simulink model "Harness_computeBaseFourierSubset"  (R2017b)
settings: Solver=FixedStepDiscrete  StartTime=0.0  StopTime=simulationTime/3  RelTol=1e-3
InitFcn:
  | referenceVector = getBaseFourierSubset(nRecurrences, nFilters);
undefined symbols (not defined in the file): nFilters, oversamplingFactor, sizeRAMs
settings Model: Creator=pnowodzi  LastModifiedBy=pnowodzi
settings DataIOCC: ExternalInput=tb_computeBaseFourierSubset.getElement('phaseIncrement'),tb_computeBaseFourierSubset.getElement('startAnalysis'),tb_computeBaseFourierSubset.getElement('syncRecurrence'),tb_computeBaseFourierSubset.getElement('nRecurrences')  LimitDataPoints=on  LoadExternalInput=on  SaveTime=off
settings OptimizationCC: BlockReduction=off  ConditionallyExecuteInputs=off  DefaultParameterBehavior=Inlined  LifeSpan=inf
settings DebuggingCC: AlgebraicLoopMsg=error  SingleTaskRateTransMsg=error  AllowSymbolicDim=off  StrictBusMsg=ErrorOnBusTreatedAsVector  SFUnexpectedBacktrackingDiag=warning  SFNoUnconditionalDefaultTransitionDiag=warning  SFExecutionAtInitializationDiag=none
settings HardwareCC: ProdBitPerPointer=32  ProdBitPerSizeT=32  ProdBitPerPtrDiffT=32  ProdLargestAtomicFloat=None  ProdIntDivRoundTo=Undefined  ProdEndianess=Unspecified  ProdWordSize=32  ProdHWDeviceType=ASIC/FPGA->ASIC/FPGA  ProdEqTarget=off
settings CodeAppCC: StateflowObjectComments=on
settings GRTTargetCC: TargetLangStandard=C89/C90 (ANSI)  GeneratePreprocessorConditionals=Disable all
settings ConfigComp: CovScope=ReferencedModels  CovMetricSettings=dw  CovHtmlReporting=on  CovSaveCumulativeToWorkspaceVar=on  CovSaveSingleToWorkspaceVar=on  CovExternalEMLEnable=off  CovSFcnEnable=off

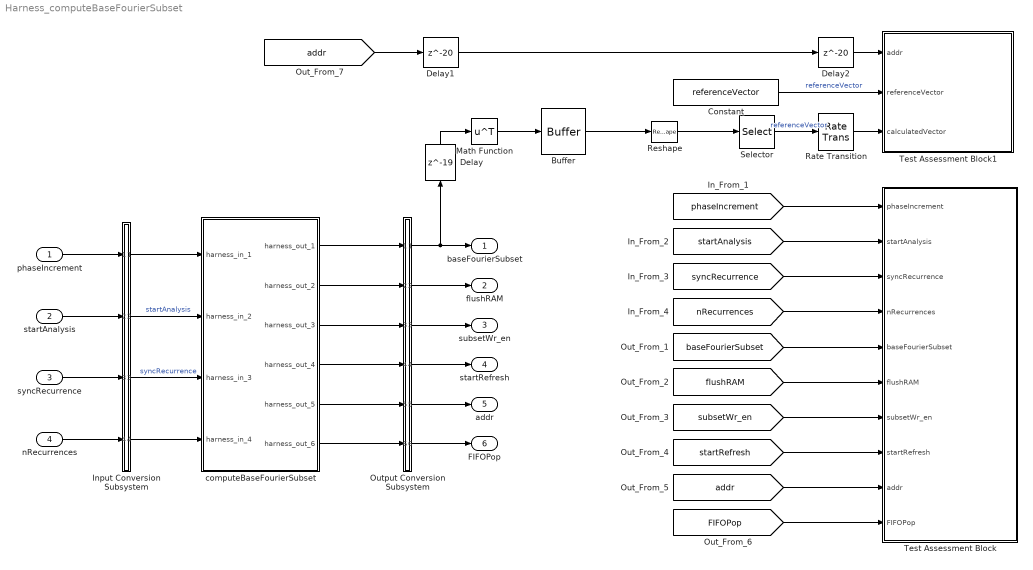
== system Harness_computeBaseFourierSubset ==
  phaseIncrement : Inport  OutDataTypeStr=fixdt('ufix16_En20')  PortDimensions=[1]  SampleTime=4e-09  Interpolate=off
  startAnalysis : Inport  Port=2  OutDataTypeStr=boolean  PortDimensions=[1]  SampleTime=4e-09
  syncRecurrence : Inport  Port=3  OutDataTypeStr=boolean  PortDimensions=[1]  SampleTime=4e-09
  nRecurrences : Inport  Port=4  OutDataTypeStr=fixdt('ufix10')  PortDimensions=[1]  SampleTime=4e-09  Interpolate=off
  Buffer : Buffer  N=oversamplingFactor  OutputFrames=off
  Constant : Constant  Value=referenceVector  SampleTime=-1
  Delay : Delay  DelayLength=19
  Delay1 : Delay  DelayLength=20
  Delay2 : Delay  DelayLength=20
  Input Conversion Subsystem : Subsystem  Tag=__SLT_ICS__  Description=|
      | Signal spec.
      | and routing
      settings: AttributesFormatString=%<Description>
  Math Function : Math  Operator=transpose  SaturateOnIntegerOverflow=on
  Output Conversion Subsystem : Subsystem  Tag=__SLT_OCS__  Description=|
      | Signal spec.
      | and routing
      settings: AttributesFormatString=%<Description>
  Rate Transition : RateTransition
  Reshape : Reshape
  Selector : Selector  InputPortWidth=ceil(nFilters/2/oversamplingFactor)*oversamplingFactor  IndexOptions=Index vector (dialog)  Indices=(1:floor((nFilters-1)/2 + 1))  OutputSizes=1
  Test Assessment Block : Test Sequence  Tag=__SLT_ASMT__  TreatAsAtomicUnit=on
  Test Assessment Block1 : Test Sequence  Tag=__SLT_ASMT__  TreatAsAtomicUnit=on
  computeBaseFourierSubset : Subsystem  Tag=__SL_testing_harness_stub_
  baseFourierSubset : Outport  OutDataTypeStr=single  PortDimensions=[6, 1]
      settings: SignalType=complex
  flushRAM : Outport  Port=2  OutDataTypeStr=boolean  PortDimensions=[1]
  subsetWr_en : Outport  Port=3  OutDataTypeStr=boolean  PortDimensions=[1]
  startRefresh : Outport  Port=4  OutDataTypeStr=boolean  PortDimensions=[1]
  addr : Outport  Port=5  OutDataTypeStr=uint8  PortDimensions=[1]
  FIFOPop : Outport  Port=6  OutDataTypeStr=boolean  PortDimensions=[1]
  wires:
  [phaseIncrement] -> Test Assessment Block/1(phaseIncrement)
  [startAnalysis] -> Test Assessment Block/2(startAnalysis)
  [syncRecurrence] -> Test Assessment Block/3(syncRecurrence)
  [nRecurrences] -> Test Assessment Block/4(nRecurrences)
  [baseFourierSubset] -> Test Assessment Block/5(baseFourierSubset)
  [flushRAM] -> Test Assessment Block/6(flushRAM)
  [subsetWr_en] -> Test Assessment Block/7(subsetWr_en)
  [startRefresh] -> Test Assessment Block/8(startRefresh)
  [addr] -> Test Assessment Block/9(addr)
  [FIFOPop] -> Test Assessment Block/10(FIFOPop)
  phaseIncrement/1 -> Input Conversion Subsystem/1(Inport_1)
  startAnalysis/1 -> Input Conversion Subsystem/2(Inport_2)
  syncRecurrence/1 -> Input Conversion Subsystem/3(Inport_3)
  Output Conversion Subsystem/1(Outport_1) -> Delay/1, baseFourierSubset/1
  Output Conversion Subsystem/2(Outport_2) -> flushRAM/1
  Output Conversion Subsystem/3(Outport_3) -> subsetWr_en/1
  Output Conversion Subsystem/4(Outport_4) -> startRefresh/1
  Output Conversion Subsystem/5(Outport_5) -> addr/1
  Output Conversion Subsystem/6(Outport_6) -> FIFOPop/1
  Input Conversion Subsystem/1(Outport_1) -> computeBaseFourierSubset/1(harness_in_1)
  Input Conversion Subsystem/2(Outport_2) -> computeBaseFourierSubset/2(harness_in_2)  "startAnalysis"
  Input Conversion Subsystem/3(Outport_3) -> computeBaseFourierSubset/3(harness_in_3)  "syncRecurrence"
  Input Conversion Subsystem/4(Outport_4) -> computeBaseFourierSubset/4(harness_in_4)
  computeBaseFourierSubset/1(harness_out_1) -> Output Conversion Subsystem/1(Inport_1)
  computeBaseFourierSubset/2(harness_out_2) -> Output Conversion Subsystem/2(Inport_2)
  computeBaseFourierSubset/3(harness_out_3) -> Output Conversion Subsystem/3(Inport_3)
  computeBaseFourierSubset/4(harness_out_4) -> Output Conversion Subsystem/4(Inport_4)
  computeBaseFourierSubset/6(harness_out_6) -> Output Conversion Subsystem/6(Inport_6)
  Reshape/1 -> Selector/1
  nRecurrences/1 -> Input Conversion Subsystem/4(Inport_4)
  Constant/1 -> Test Assessment Block1/2(referenceVector)  "referenceVector"
  Math Function/1 -> Buffer/1
  Delay/1 -> Math Function/1
  Buffer/1 -> Reshape/1
  Selector/1 -> Rate Transition/1  "referenceVector"
  [addr] -> Delay1/1
  computeBaseFourierSubset/5(harness_out_5) -> Output Conversion Subsystem/5(Inport_5)
  Delay1/1 -> Delay2/1
  Rate Transition/1 -> Test Assessment Block1/3(calculatedVector)
  Delay2/1 -> Test Assessment Block1/1(addr)

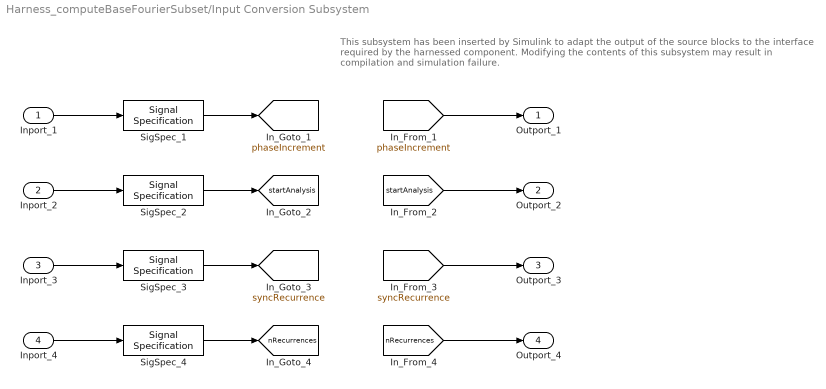
== system Harness_computeBaseFourierSubset/Input Conversion Subsystem ==
  note: This subsystem has been inserted by Simulink to adapt the output of the source blocks to the interface required by the harnessed component.
      |  Modifying the contents of this subsystem may result in compilation and simulation failure.
  Inport_1 : Inport
  Inport_2 : Inport  Port=2
  Inport_3 : Inport  Port=3
  Inport_4 : Inport  Port=4
  SigSpec_1 : SignalSpecification  OutDataTypeStr=fixdt('ufix16_En20')  Dimensions=[1]  SampleTime=4e-09
  SigSpec_2 : SignalSpecification  OutDataTypeStr=boolean  Dimensions=[1]  SampleTime=4e-09
  SigSpec_3 : SignalSpecification  OutDataTypeStr=boolean  Dimensions=[1]  SampleTime=4e-09
  SigSpec_4 : SignalSpecification  OutDataTypeStr=fixdt('ufix10')  Dimensions=[1]  SampleTime=4e-09
  Outport_1 : Outport
  Outport_2 : Outport  Port=2
  Outport_3 : Outport  Port=3
  Outport_4 : Outport  Port=4
  tag scope: nRecurrences=global, phaseIncrement=global, startAnalysis=global, syncRecurrence=global
  wires:
  [phaseIncrement] -> Outport_1/1
  SigSpec_1/1 -> [phaseIncrement]
  Inport_1/1 -> SigSpec_1/1
  [startAnalysis] -> Outport_2/1
  SigSpec_2/1 -> [startAnalysis]
  Inport_2/1 -> SigSpec_2/1
  [syncRecurrence] -> Outport_3/1
  SigSpec_3/1 -> [syncRecurrence]
  Inport_3/1 -> SigSpec_3/1
  [nRecurrences] -> Outport_4/1
  SigSpec_4/1 -> [nRecurrences]
  Inport_4/1 -> SigSpec_4/1

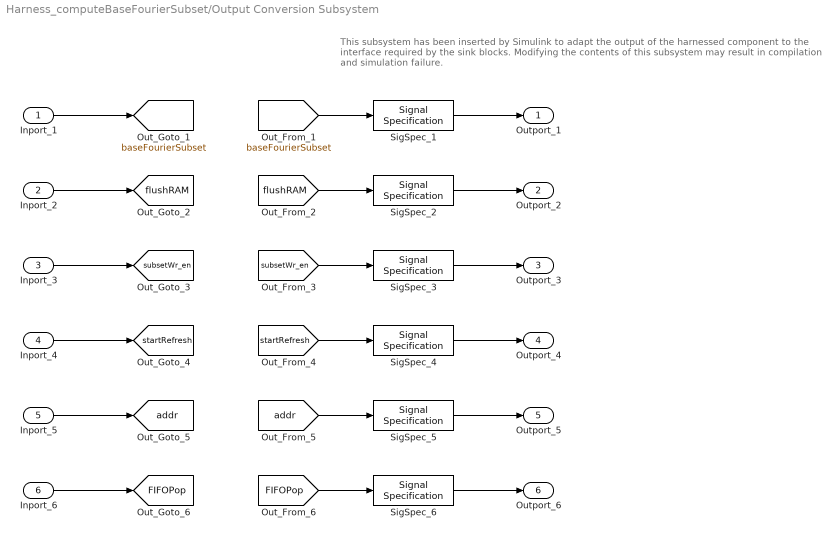
== system Harness_computeBaseFourierSubset/Output Conversion Subsystem ==
  note: This subsystem has been inserted by Simulink to adapt the output of the harnessed component to the interface required by the sink blocks.
      |  Modifying the contents of this subsystem may result in compilation and simulation failure.
  Inport_1 : Inport
  Inport_2 : Inport  Port=2
  Inport_3 : Inport  Port=3
  Inport_4 : Inport  Port=4
  Inport_5 : Inport  Port=5
  Inport_6 : Inport  Port=6
  SigSpec_1 : SignalSpecification  OutDataTypeStr=single  Dimensions=[6, 1]  SampleTime=4e-09
      settings: SignalType=complex
  SigSpec_{2..4,6} (4 alike) : SignalSpecification  OutDataTypeStr=boolean  Dimensions=[1]  SampleTime=4e-09
  SigSpec_5 : SignalSpecification  OutDataTypeStr=uint8  Dimensions=[1]  SampleTime=4e-09
  Outport_1 : Outport
  Outport_2 : Outport  Port=2
  Outport_3 : Outport  Port=3
  Outport_4 : Outport  Port=4
  Outport_5 : Outport  Port=5
  Outport_6 : Outport  Port=6
  tag scope: FIFOPop=global, addr=global, baseFourierSubset=global, flushRAM=global, startRefresh=global, subsetWr_en=global
  wires:
  Inport_1/1 -> [baseFourierSubset]
  [baseFourierSubset] -> SigSpec_1/1
  SigSpec_1/1 -> Outport_1/1
  Inport_2/1 -> [flushRAM]
  [flushRAM] -> SigSpec_2/1
  SigSpec_2/1 -> Outport_2/1
  Inport_3/1 -> [subsetWr_en]
  [subsetWr_en] -> SigSpec_3/1
  SigSpec_3/1 -> Outport_3/1
  Inport_4/1 -> [startRefresh]
  [startRefresh] -> SigSpec_4/1
  SigSpec_4/1 -> Outport_4/1
  Inport_5/1 -> [addr]
  [addr] -> SigSpec_5/1
  SigSpec_5/1 -> Outport_5/1
  Inport_6/1 -> [FIFOPop]
  [FIFOPop] -> SigSpec_6/1
  SigSpec_6/1 -> Outport_6/1

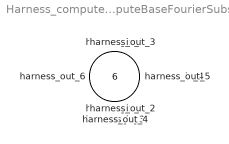
== system Harness_computeBaseFourierSubset/computeBaseFourierSubset ==
  harness_in_1 : Inport
  harness_in_2 : Inport  Port=2
  harness_in_3 : Inport  Port=3
  harness_in_4 : Inport  Port=4
  harness_out_1 : Outport
  harness_out_2 : Outport  Port=2
  harness_out_3 : Outport  Port=3
  harness_out_4 : Outport  Port=4
  harness_out_5 : Outport  Port=5
  harness_out_6 : Outport  Port=6

== stateflow chart Harness_computeBaseFourierSubset/Test Assessment Block ==
  settings: stateMachineType=SIMPLIFIED_MACHINE
  state Run
    state step_1_1
    state step_1_2
    (default) -> (junction 22)
    Run -> (junction 22)
    (junction 22) -> (junction 23) [order 1] : [t < 5]
    (junction 23) -> step_1_1 [order 1] : [~in(step_1_1)]
    (junction 23) -> (junction 26) [order 2]
    (junction 31) -> (junction 32)
    (junction 32) -> step_1_2 [order 1] : [~in(step_1_2)]
    (junction 32) -> (junction 35) [order 2]
    (junction 22) -> (junction 31) [order 2]
  (default) -> Run
  data: phaseIncrement input fixdt('ufix16_En20') size=[1]; startAnalysis input boolean size=[1]; syncRecurrence input boolean size=[1]; nRecurrences input fixdt('ufix10') size=[1]; baseFourierSubset input single size=[6, 1]; flushRAM input boolean size=[1]; subsetWr_en input boolean size=[1]; startRefresh input boolean size=[1]; addr input uint8 size=[1]; FIFOPop input boolean size=[1]

== stateflow chart Harness_computeBaseFourierSubset/Test Assessment Block1 ==
  settings: stateMachineType=SIMPLIFIED_MACHINE
  state Run
    tolerance = 1e-6;
    state baseFourierSubsetVerification
      verify(all(referenceVector - tolerance <= calculatedVector)   &&  all(referenceVector + tolerance >= calculatedVector));
    state idle
    (junction 70) -> baseFourierSubsetVerification [order 1] : [~in(baseFourierSubsetVerification)]
    (junction 81) -> (junction 70) [order 1] : [addr == sizeRAMs-1
        | ]
    (junction 70) -> (junction 73) [order 2]
    (junction 101) -> (junction 102)
    (junction 102) -> idle [order 1] : [~in(idle)]
    (junction 81) -> (junction 101) [order 2]
    (junction 102) -> (junction 105) [order 2]
    (default) -> (junction 81)
    Run -> (junction 81)
  (default) -> Run
  data: addr input; referenceVector input; calculatedVector input; nFilters parameter; sizeRAMs parameter; tolerance local
